simulink model "testingBagFile"  (R2025a)
settings: Solver=VariableStepAuto  StartTime=0.0  StopTime=1600  RelTol=1e-3
undefined symbols (not defined in the file): SampleTime
libraries: simulink_extras x2, simulink x2, eeGeneralControl x2
settings Model: Creator=Viktor Traktor  LastModifiedBy=eliasalbag

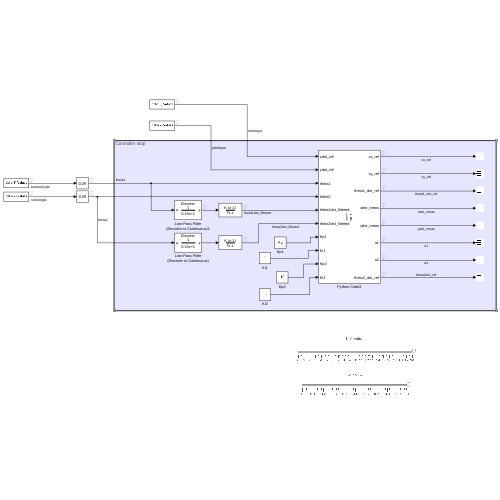
[thumbnail: Simulink's stored preview of the top-level diagram]
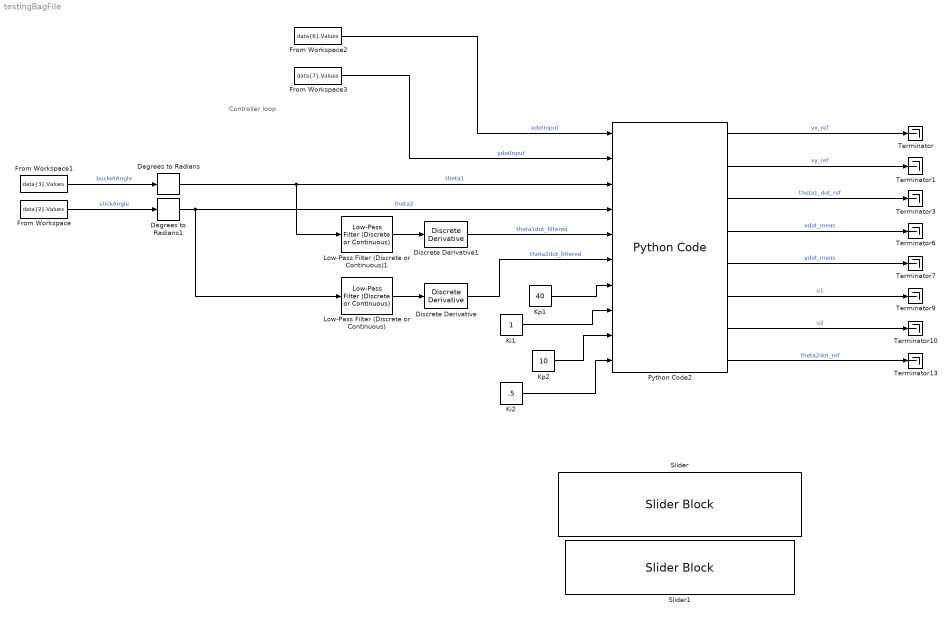
== system testingBagFile ==
  note: Controller loop
  Degrees to Radians : simulink_extras/Transformations/Degrees to Radians
  Degrees to Radians1 : simulink_extras/Transformations/Degrees to Radians
  Discrete Derivative : simulink/Discrete/Discrete Derivative  gainval=1.0  ICPrevScaledInput=0.0  OutMin=[]  OutMax=[]  OutDataType=fixdt(1, 16)  OutScaling=2^-10  DoSatur=off
  Discrete Derivative1 : simulink/Discrete/Discrete Derivative  gainval=1.0  ICPrevScaledInput=0.0  OutMin=[]  OutMax=[]  OutDataType=fixdt(1, 16)  OutScaling=2^-10  DoSatur=off
  From Workspace : FromWorkspace  VariableName=data{2}.Values
  From Workspace1 : FromWorkspace  VariableName=data{3}.Values
  From Workspace2 : FromWorkspace  VariableName=data{6}.Values
  From Workspace3 : FromWorkspace  VariableName=data{7}.Values
  Ki1 : Constant
  Ki2 : Constant  Value=.5
  Kp1 : Constant  Value=40
  Kp2 : Constant  Value=10
  Low-Pass Filter (Discrete or Continuous) : eeGeneralControl/Low-Pass Filter (Discrete or Continuous)  K=1  T=.15  B=inf  A=-inf  init_option=Inherited from block input  x0=0  Ts=0.1
  Low-Pass Filter (Discrete or Continuous)1 : eeGeneralControl/Low-Pass Filter (Discrete or Continuous)  K=1  T=.15  B=inf  A=-inf  init_option=Inherited from block input  x0=0  Ts=0.1
  Python Code2 : PythonCode  OutputCode=|  SampleTime=SampleTime  max_joint_vel1=.5  max_joint_vel2=.5  SampleTime=.1
      | import numpy as np
      | 
      | # Inputs:
      | #   xdot_ref, ydot_ref in [-1, 1]   (joystick commands, normalized)
      | #   theta1, theta2 [rad]            (joint angles)
      | #   max_joint_vel1, max_joint_vel2  [rad/s]
      | #
      | # Outputs:
      | #   u1, u2 in [-100, 100]           (valve commands)
      | 
      | 
      | # -------------------------------------------------------------------
      | # Constants
      | # -------------------------------------------------------------------
      | DT = 0.1  # time step [s]
      | 
      | VX_MAX = 0.05  # max Cartesian speed along x [m/s]
      | VY_MAX = 0.05 # max Cartesian speed along y [m/s]
      | 
      | AXIS_DEADZONE_NORM = 0.05   # joystick deadzone in normalized units [-1, 1]
      | 
      | M0 = 0.08      # shaping deadzone
      | P_SHAPE = 2.0  # shaping exponent
      | 
      | # Link lengths [m]
      | L1 = 1903.392e-3
      | L2 = 1351.485e-3
      | L3 = 590.267e-3  # not using the bucket angle here
      | 
      | # Joint-space PID gains
      | #Kp = .7
      | #Ki = 0.3
      | Kd1 = 0.0
      | Kd2 = 0.0
      | 
      | # -------------------------------------------------------------------
      | # 1) Joystick -> Cartesian velocity reference (axis-locked)
      | # -------------------------------------------------------------------
      | 
      | # default (deadzone or no input)
      | vx_ref = 0.0
      | vy_ref = 0.0
      | 
      | if not (abs(xdot_ref) <= AXIS_DEADZONE_NORM and abs(ydot_ref) <= AXIS_DEADZONE_NORM):
      | 
      |     # Decide dominant axis: X-mode or Y-mode
      |     if abs(xdot_ref) > abs(ydot_ref):
      |         # X-mode
      |         vel_ref = xdot_ref
      |         v_max = VX_MAX
      | 
      |         if abs(vel_ref) > AXIS_DEADZONE_NORM:
      |             # sign
      |             sign = 1.0 if vel_ref >= 0.0 else -1.0
      |             # normalize magnitude into [0,1] after deadzone
      |             mag_norm = (abs(vel_ref) - AXIS_DEADZONE_NORM) / (1.0 - AXIS_DEADZONE_NORM)
      | 
      |             # shaping
      |             if mag_norm <= M0:
      |                 f = 0.0
      |             else:
      |                 r = (mag_norm - M0) / (1.0 - M0)
      |                 f = r ** P_SHAPE
      | 
      |             vx_ref = sign * v_max * f
      |             vy_ref = 0.0
      | 
      |     else:
      |         # Y-mode
      |         vel_ref = ydot_ref
      |         v_max = VY_MAX
      | 
      |         if abs(vel_ref) > AXIS_DEADZONE_NORM:
      |             sign = 1.0 if vel_ref >= 0.0 else -1.0
      |             mag_norm = (abs(vel_ref) - AXIS_DEADZONE_NORM) / (1.0 - AXIS_DEADZONE_NORM)
      | 
      |             if mag_norm <= M0:
      |                 f = 0.0
      |             else:
      |                 r = (mag_norm - M0) / (1.0 - M0)
      |                 f = r ** P_SHAPE
      | 
      |             vy_ref = sign * v_max * f
      |             vx_ref = 0.0
      | 
      | xydot_ref = np.array([vx_ref, vy_ref])
      | 
      | # -------------------------------------------------------------------
      | # 2) Jacobian and joint velocity reference (IK)
      | # -------------------------------------------------------------------
      | 
      | J11 = -L1 * np.sin(theta1) - L2 * np.sin(theta1 + theta2)
      | J12 = -L2 * np.sin(theta1 + theta2)
      | J21 =  L1 * np.cos(theta1) + L2 * np.cos(theta1 + theta2)
      | J22 =  L2 * np.cos(theta1 + theta2)
      | 
      | J = np.array([[J11, J12],
      |               [J21, J22]])
      | 
      | Jpinv = np.linalg.pinv(J)
      | 
      | theta_dot_ref_vec = Jpinv @ xydot_ref
      | theta1_dot_ref = float(theta_dot_ref_vec[0])
      | theta2_dot_ref = float(theta_dot_ref_vec[1])
      | 
      | theta1_dot_ref = float(np.clip(theta1_dot_ref, -max_joint_vel1, max_joint_vel1))
      | theta2_dot_ref = float(np.clip(theta2_dot_ref, -max_joint_vel2, max_joint_vel2))
      | theta_dot_ref_vec = np.array([theta1_dot_ref, theta2_dot_ref])
      | 
      | 
      | # -------------------------------------------------------------------
      | # 3) Measured joint velocities 
      | # -------------------------------------------------------------------
      | 
      | '''
      | if theta1_prev is None:
      |     theta1_prev = theta1
      | if theta2_prev is None:
      |     theta2_prev = theta2
      | 
      | theta1dot_meas = (theta1 - theta1_prev) / DT
      | theta2dot_meas = (theta2 - theta2_prev) / DT
      | 
      | theta1_prev = theta1
      | theta2_prev = theta2
      | 
      | '''
      | 
      | thetadot_meas_vec = np.array([theta1dot_filtered, theta2dot_filtered])
      | 
      | 
      | 
      | 
      | # -------------------------------------------------------------------
      | # Logg detta i Simulink för: Cartesian measured velocity & error
      | # -------------------------------------------------------------------
      | 
      | xydot_meas = J @ thetadot_meas_vec
      | xdot_meas = float(xydot_meas[0])
      | ydot_meas = -float(xydot_meas[1])
      | 
      | xydot_error = xydot_ref - xydot_meas
      | xdot_error = float(xydot_error[0])
      | ydot_error = float(xydot_error[1])
      | 
      | 
      | # -------------------------------------------------------------------
      | # 4) Joint velocity error (for joint-space PID)
      | # -------------------------------------------------------------------
      | 
      | thetadot_error = theta_dot_ref_vec - thetadot_meas_vec
      | theta1dot_error = thetadot_error[0]
      | theta2dot_error = thetadot_error[1]
      | 
      | 
      | # -------------------------------------------------------------------
      | # 5) Integral term (trapezoidal)
      | # -------------------------------------------------------------------
      | 
      | if thetadot1_error_prev is None:
      |     thetadot1_error_prev = 0.0
      | if thetadot2_error_prev is None:
      |     thetadot2_error_prev = 0.0
      | 
      | theta1dot_error_integral = (
      |     (theta1dot_error + thetadot1_error_prev) * DT / 2.0
      |     + thetadot1_error_integral_prev
      | )
      | theta2dot_error_integral = (
      |     (theta2dot_error + thetadot2_error_prev) * DT / 2.0
      |     + thetadot2_error_integral_prev
      | )
      | 
      | thetadot1_error_integral_prev = theta1dot_error_integral
      | thetadot2_error_integral_prev = theta2dot_error_integral
      | 
      | thetadot_error_integral = np.array([
      |     theta1dot_error_integral,
      |     theta2dot_error_integral
      | ])
      | 
      | 
      | # -------------------------------------------------------------------
      | # 6) Derivative term
      | # -------------------------------------------------------------------
      | 
      | theta1dot_error_derivative = (theta1dot_error - thetadot1_error_prev) / DT
      | theta2dot_error_derivative = (theta2dot_error - thetadot2_error_prev) / DT
      | 
      | thetadot_error_derivative = np.array([
      |     theta1dot_error_derivative,
      |     theta2dot_error_derivative
      | ])
      | 
      | thetadot1_error_prev = theta1dot_error
      | thetadot2_error_prev = theta2dot_error
      | 
      | 
      | u1 = -(Kp1*theta1dot_error + Ki1*theta1dot_error_integral + Kd1*theta1dot_error_derivative)
      | u2 = (Kp2*theta2dot_error + Ki2*theta2dot_error_integral + Kd2*theta2dot_error_derivative)
  Slider : SliderBlock  ScaleMax=20
  Slider1 : SliderBlock  ScaleMax=1
  Terminator{,1,3,6..7,9..10,13} (8 alike) : Terminator
  wires:
  Discrete Derivative/1 -> Python Code2/6  "theta2dot_filtered"
  Degrees to Radians1/1 -> Low-Pass Filter (Discrete or Continuous)/1, Python Code2/4  "theta2"
  Discrete Derivative1/1 -> Python Code2/5  "theta1dot_filtered"
  Low-Pass Filter (Discrete or Continuous)1/1 -> Discrete Derivative1/1
  Python Code2/2 -> Terminator1/1  "vy_ref"
  Python Code2/1 -> Terminator/1  "vx_ref"
  Python Code2/3 -> Terminator3/1  "theta1_dot_ref"
  Degrees to Radians/1 -> Low-Pass Filter (Discrete or Continuous)1/1, Python Code2/3  "theta1"
  Python Code2/5 -> Terminator7/1  "ydot_meas"
  Kp1/1 -> Python Code2/7
  Low-Pass Filter (Discrete or Continuous)/1 -> Discrete Derivative/1
  Python Code2/8 -> Terminator13/1  "theta2dot_ref"
  Ki1/1 -> Python Code2/8
  Python Code2/6 -> Terminator9/1  "u1"
  Python Code2/4 -> Terminator6/1  "xdot_meas"
  Python Code2/7 -> Terminator10/1  "u2"
  From Workspace/1 -> Degrees to Radians1/1  "stickAngle"
  From Workspace1/1 -> Degrees to Radians/1  "bucketAngle"
  From Workspace3/1 -> Python Code2/2  "ydotInput"
  From Workspace2/1 -> Python Code2/1  "xdotInput"
  Kp2/1 -> Python Code2/9
  Ki2/1 -> Python Code2/10
